simulink model "sim2_2_2"  (R2017b)
settings: Solver=ode5  StartTime=0.0  StopTime=10  FixedStep=0.001  RelTol=1e-3
settings Model: Creator=kiran  LastModifiedBy=kiran

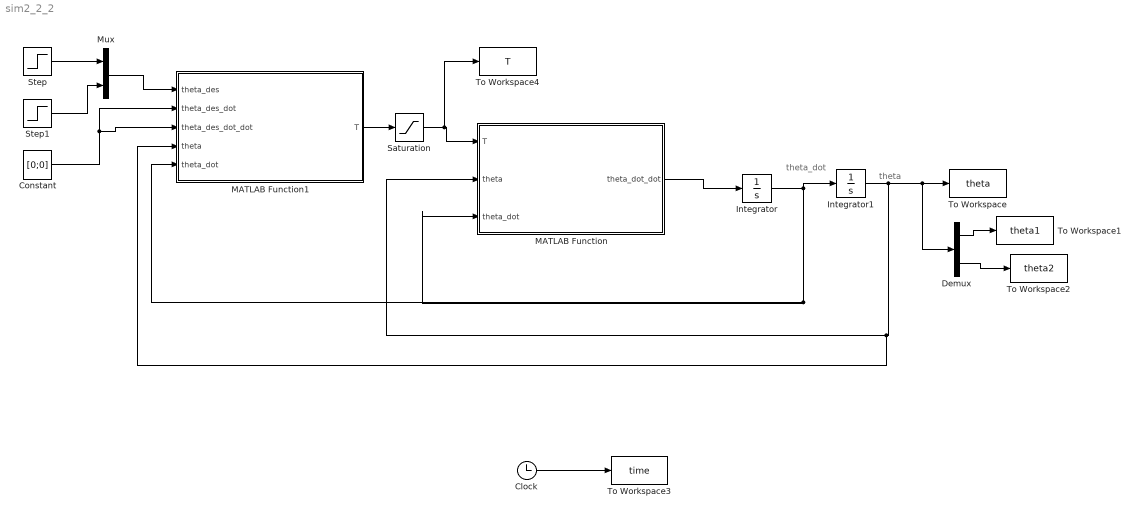
== system sim2_2_2 ==
  note: theta
  note: theta_dot
  Clock : Clock
  Constant : Constant  Value=[0;0]
  Demux : Demux  Outputs=2
  Integrator : Integrator  InitialCondition=[0;0]
  Integrator1 : Integrator  InitialCondition=[-pi/2;0]
  MATLAB Function : MATLAB Function  TreatAsAtomicUnit=on
  MATLAB Function1 : MATLAB Function  TreatAsAtomicUnit=on
  Mux : Mux  Inputs=2
  Saturation : Saturate  UpperLimit=5  LowerLimit=-5
  Step : Step  Time=5  After=-3*pi/4  SampleTime=0
  Step1 : Step  Time=5  After=pi/4  SampleTime=0
  To Workspace : ToWorkspace  VariableName=theta  SampleTime=-1
  To Workspace1 : ToWorkspace  VariableName=theta1  SampleTime=-1
  To Workspace2 : ToWorkspace  VariableName=theta2  SampleTime=-1
  To Workspace3 : ToWorkspace  VariableName=time  SampleTime=-1
  To Workspace4 : ToWorkspace  VariableName=T  SampleTime=-1
  wires:
  MATLAB Function/1(theta_dot_dot) -> Integrator/1
  Integrator/1 -> MATLAB Function1/5(theta_dot), MATLAB Function/3(theta_dot), Integrator1/1
  Integrator1/1 -> MATLAB Function1/4(theta), MATLAB Function/2(theta), Demux/1, To Workspace/1
  Demux/1 -> To Workspace1/1
  Demux/2 -> To Workspace2/1
  Clock/1 -> To Workspace3/1
  Saturation/1 -> To Workspace4/1, MATLAB Function/1(T)
  MATLAB Function1/1(T) -> Saturation/1
  Mux/1 -> MATLAB Function1/1(theta_des)
  Step/1 -> Mux/1
  Step1/1 -> Mux/2
  Constant/1 -> MATLAB Function1/3(theta_des_dot_dot), MATLAB Function1/2(theta_des_dot)

== matlab function sim2_2_2/MATLAB Function1 ==
  data: theta_des input; theta_des_dot input; theta_des_dot_dot input; T output; theta input; theta_dot input
function T = fcn3(theta_des,theta_des_dot,theta_des_dot_dot, theta, theta_dot)
l1 =0.5;    %m
l2 = 0.3;   %m
r1 = 0.25;  %m
r2 = 0.15;  %m
m1 = 0.5;   %kg
m2 = 0.3;   %kg
I1 = 0.0104;%kg-m^2
I2 = 0.0022;%kg-m^2
c1 = 0;     %N.m.s/rad
c2 = 0;     %N.m.s/rad
g = 9.81;   %m/s^2

alpha = I1+I2+m1*r1^2+m2*(l1^2+r2^2);
beta = m2*l1*r2;
gamma = I2+m2*r2^2;

theta1 = theta(1);
theta2 = theta(2);
theta1_dot = theta_dot(1);
theta2_dot = theta_dot(2);

M =[alpha+2*beta.*cos(theta2) gamma+beta.*cos(theta2); gamma+beta.*cos(theta2) gamma];
C = [c1-beta.*theta2_dot.*sin(theta2) -beta.*(theta1_dot+theta2_dot).*sin(theta2); beta*theta1_dot.*sin(theta2) c2];
N = [(m1*r1+m2*l1)*g.*cos(theta1)+m2*r2*g.*cos(theta1+theta2); m2*r2*g.*cos(theta1+theta2)];

lambda=10;

K1=[2*lambda; 2*lambda];
K2=[lambda^2;lambda^2];

e=theta_des-theta;

e_dot=theta_des_dot-theta_dot;

e_dot_dot=-K1.*e_dot-K2.*e;

T=M*theta_des_dot_dot-M*e_dot_dot+C*theta_dot+N;

end

== matlab function sim2_2_2/MATLAB Function ==
  data: T input; theta_dot_dot output; theta input; theta_dot input
function theta_dot_dot = fcn(T,theta,theta_dot)
l1 =0.5;    %m
l2 = 0.3;   %m
r1 = 0.25;  %m
r2 = 0.15;  %m
m1 = 0.5;   %kg
m2 = 0.3;   %kg
I1 = 0.0104;%kg-m^2
I2 = 0.0022;%kg-m^2
c1 = 0;     %N.m.s/rad
c2 = 0;     %N.m.s/rad
g = 9.81;   %m/s^2

alpha = I1+I2+m1*r1^2+m2*(l1^2+r2^2);
beta = m2*l1*r2;
gamma = I2+m2*r2^2;

theta1 = theta(1);
theta2 = theta(2);
theta1_dot = theta_dot(1);
theta2_dot = theta_dot(2);

M =[alpha+2*beta.*cos(theta2) gamma+beta.*cos(theta2); gamma+beta.*cos(theta2) gamma];
C = [c1-beta.*theta2_dot.*sin(theta2) -beta.*(theta1_dot+theta2_dot).*sin(theta2); beta*theta1_dot.*sin(theta2) c2];
N = [(m1*r1+m2*l1)*g.*cos(theta1)+m2*r2*g.*cos(theta1+theta2); m2*r2*g.*cos(theta1+theta2)];

theta_dot_dot = inv(M)*(T-C*theta_dot-N);
end
